simulink model "FSK"  (Simulink 7.9)
settings: Solver=ode45  StartTime=0.0  StopTime=100  RelTol=1e-3
libraries: commrandsrc2 x1, simulink x1, commsynccomp2 x1
settings Model: Creator=usuario  LastModifiedBy=davito
settings OptimizationCC: InitFltsAndDblsToZero=on
settings DebuggingCC: SaveWithParameterizedLinksMsg=none  SignalResolutionControl=TryResolveAllWithWarning  MultiTaskDSMMsg=warning  MultiTaskCondExecSysMsg=none  FcnCallInpInsideContextMsg=Use local settings  StrictBusMsg=Warning
settings RTWCC: IncludeERTFirstTime=on
settings GRTTargetCC: TargetFcnLib=ansi_tfl_tmw.mat  CombineOutputUpdateFcns=off  GRTInterface=on

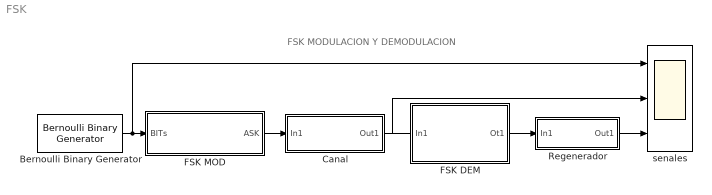
== system FSK ==
  note: FSK MODULACION Y DEMODULACION
  Bernoulli Binary Generator : commrandsrc2/Bernoulli Binary Generator  P=0.3  seed=61  Ts=5  frameBased=off  sampPerFrame=1  orient=off  outDataType=double
  Canal : Subsystem
  FSK DEM : Subsystem
  FSK MOD : Subsystem
  Regenerador : Subsystem
  senales : Scope  NumInputPorts=3
      settings: YMin=-5~-5~-5  YMax=5~5~5
  wires:
  Bernoulli Binary Generator/1 -> FSK MOD/1(BITs), senales/1
  FSK MOD/1(ASK) -> Canal/1(In1)
  FSK DEM/1(Ot1) -> Regenerador/1(In1)
  Canal/1(Out1) -> FSK DEM/1(In1), senales/2
  Regenerador/1(Out1) -> senales/3

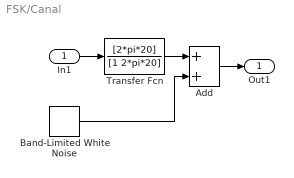
== system FSK/Canal ==
  In1 : Inport
  Add : Sum
  Band-Limited White Noise : simulink/Sources/Band-Limited White Noise  SystemSampleTime=-1  Cov=[0.002]  Ts=1  seed=[23341]
  Transfer Fcn : TransferFcn  Numerator=[2*pi*20]  Denominator=[1 2*pi*20]
  Out1 : Outport
  wires:
  Transfer Fcn/1 -> Add/1
  Band-Limited White Noise/1 -> Add/2
  In1/1 -> Transfer Fcn/1
  Add/1 -> Out1/1

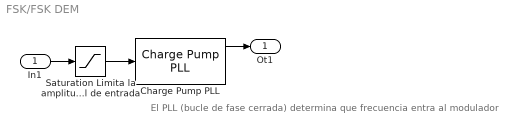
== system FSK/FSK DEM ==
  note: El PLL (bucle de fase cerrada)
      | determina que frecuencia
      | entra al modulador
  In1 : Inport
  Charge Pump PLL : commsynccomp2/Charge Pump PLL  SystemSampleTime=-1  Fn=[2*pi*1]  Fd="[1   2*pi*1]"  Kvco=4  Fc=10  Ph=0  Ac=1
  Saturation Limita la amplitud de la senal de entrada : Saturate
  Ot1 : Outport
  wires:
  In1/1 -> Saturation Limita la amplitud de la senal de entrada/1
  Charge Pump PLL/1 -> Ot1/1
  Saturation Limita la amplitud de la senal de entrada/1 -> Charge Pump PLL/1

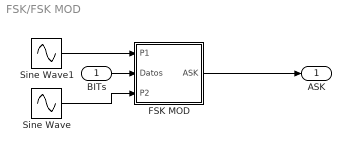
== system FSK/FSK MOD ==
  BITs : Inport
  FSK MOD : Subsystem
  Sine Wave : Sin  Frequency=2*pi*12  Samples=25  SampleTime=0.01
  Sine Wave1 : Sin  Frequency=2*pi*8  Samples=50  SampleTime=0.01
  ASK : Outport
  wires:
  BITs/1 -> FSK MOD/2(Datos)
  FSK MOD/1(ASK) -> ASK/1
  Sine Wave1/1 -> FSK MOD/1(P1)
  Sine Wave/1 -> FSK MOD/3(P2)

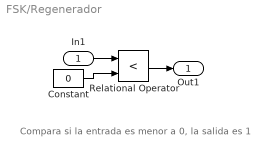
== system FSK/Regenerador ==
  note: Compara si la entrada
      | es menor a 0, la salida es 1
  In1 : Inport
  Constant : Constant  Value=0
  Relational Operator : RelationalOperator  Operator=<  OutDataTypeStr=boolean
  Out1 : Outport
  wires:
  Relational Operator/1 -> Out1/1
  In1/1 -> Relational Operator/1
  Constant/1 -> Relational Operator/2

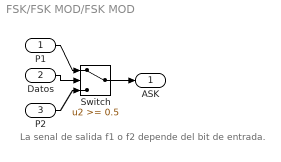
== system FSK/FSK MOD/FSK MOD ==
  note: La senal de salida f1 o f2
      | depende del bit de entrada.
  P1 : Inport
  Datos : Inport  Port=2
  P2 : Inport  Port=3
  Switch : Switch  Threshold=0.5
  ASK : Outport
  wires:
  P1/1 -> Switch/1
  Datos/1 -> Switch/2
  Switch/1 -> ASK/1
  P2/1 -> Switch/3
